simulink model "turbo"  (R2015a)
settings: Solver=ode45  StartTime=0.0  StopTime=10.0  RelTol=1e-3
libraries: commchan3 x4, commdigbbndpm3 x4, commsink2 x2, commcnvcod2 x2, commrandsrc2 x1
settings Model: Creator=jessica.c13  LastModifiedBy=jessica.c13

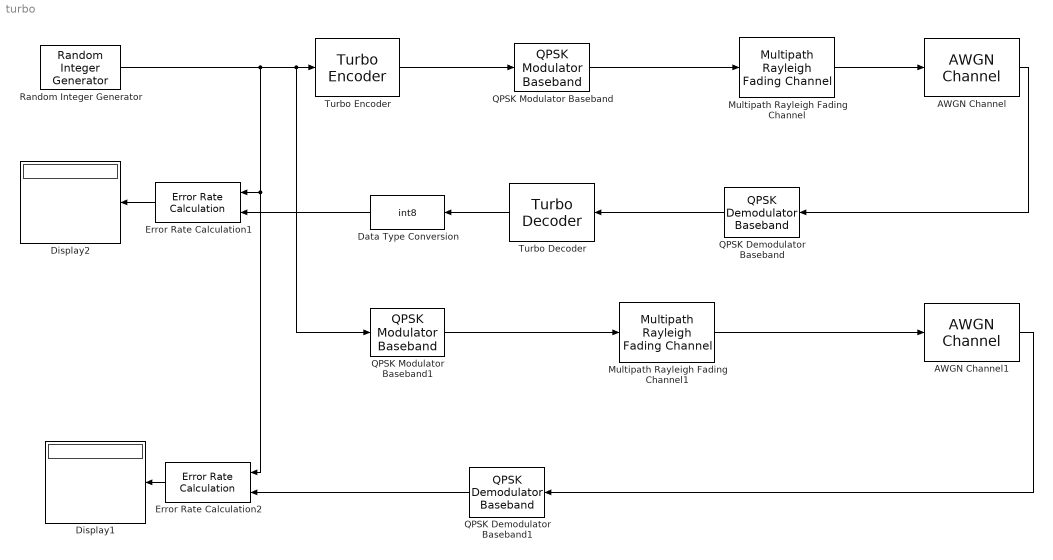
== system turbo ==
  AWGN Channel : commchan3/AWGN Channel  InputProcessing=Columns as channels (frame based)  seed=67  noiseMode="Signal to noise ratio  (Eb/No)"  EbNodB=10  EsNodB=10  SNRdB=10  bitsPerSym=1  Ps=1  Tsym=1  variance=1
  AWGN Channel1 : commchan3/AWGN Channel  InputProcessing=Columns as channels (frame based)  seed=67  noiseMode="Signal to noise ratio  (Eb/No)"  EbNodB=10  EsNodB=10  SNRdB=10  bitsPerSym=1  Ps=1  Tsym=1  variance=1
  Data Type Conversion : DataTypeConversion  OutDataTypeStr=int8
  Display1 : Display
  Display2 : Display
  Error Rate Calculation1 : commsink2/Error Rate Calculation  N=0  st_delay=0  cp_mode=Entire frame  subframe=[]  PMode=Port  WsName=e2  RsMode2=off  stop=off  numErr=100  maxBits=1e6
  Error Rate Calculation2 : commsink2/Error Rate Calculation  N=0  st_delay=0  cp_mode=Entire frame  subframe=[]  PMode=Port  WsName=e2  RsMode2=off  stop=off  numErr=100  maxBits=1e6
  Multipath Rayleigh Fading Channel : commchan3/Multipath Rayleigh Fading Channel  maxDopplerShift=40  spectrumType=Jakes  sigmaGaussian=1/sqrt(2)  coeffRounded=[1 -1.72 0.785]  freqMinMaxRJakes=[0 1]  freqMinMaxAJakes=[0 1]  sigmaGaussian1=1/sqrt(2)  sigmaGaussian2=1/sqrt(2)  centerFreqGaussian1=0.0  centerFreqGaussian2=0.0  gainGaussian1=0.5  gainGaussian2=0.5  coeffBell=9  dopplerSpectrum=doppler.jakes  pathDelays=[0 2e-6]  avgPathGaindB=[0 -3]  normalizePathGains=on  seed=73  enableProbe=0  openVisAtStart=off  outPathGains=off  outDelay=off
  Multipath Rayleigh Fading Channel1 : commchan3/Multipath Rayleigh Fading Channel  maxDopplerShift=40  spectrumType=Jakes  sigmaGaussian=1/sqrt(2)  coeffRounded=[1 -1.72 0.785]  freqMinMaxRJakes=[0 1]  freqMinMaxAJakes=[0 1]  sigmaGaussian1=1/sqrt(2)  sigmaGaussian2=1/sqrt(2)  centerFreqGaussian1=0.0  centerFreqGaussian2=0.0  gainGaussian1=0.5  gainGaussian2=0.5  coeffBell=9  dopplerSpectrum=doppler.jakes  pathDelays=[0 2e-6]  avgPathGaindB=[0 -3]  normalizePathGains=on  seed=73  enableProbe=0  openVisAtStart=off  outPathGains=off  outDelay=off
  QPSK Demodulator Baseband : commdigbbndpm3/QPSK Demodulator Baseband  Ph=pi/4  Dec=Gray  OutType=Integer  DecType=Hard decision  VarSource=Dialog  Variance=1  outDtype1=Inherit via internal rule  outDtype2=double  derotateFactorWordLen=16
  QPSK Demodulator Baseband1 : commdigbbndpm3/QPSK Demodulator Baseband  Ph=pi/4  Dec=Gray  OutType=Integer  DecType=Hard decision  VarSource=Dialog  Variance=1  outDtype1=Inherit via internal rule  outDtype2=int8  derotateFactorWordLen=16
  QPSK Modulator Baseband : commdigbbndpm3/QPSK Modulator Baseband  InType=Integer  Enc=Gray  Ph=pi/4  outDtype=double  outWordLen=16  outUDDataType=sfix(16)  outFracLenMode=Best precision  outFracLen=15
  QPSK Modulator Baseband1 : commdigbbndpm3/QPSK Modulator Baseband  InType=Integer  Enc=Gray  Ph=pi/4  outDtype=double  outWordLen=16  outUDDataType=sfix(16)  outFracLenMode=Best precision  outFracLen=15
  Random Integer Generator : commrandsrc2/Random Integer Generator  mul=2  seed=37  Ts=1/10000  frameBased=on  sampPerFrame=64  orient=off  outDataType=int8
  Turbo Decoder : commcnvcod2/Turbo Decoder  TrellisStructure=poly2trellis( 4, [ 13, 15 ], 13 )  InterleaverIndicesSource=Property  InterleaverIndices=(64:-1:1).'  Algorithm=True APP  NumScalingBits=3  NumIterations=6  SimulateUsing=Interpreted execution
  Turbo Encoder : commcnvcod2/Turbo Encoder  TrellisStructure=poly2trellis( 4, [ 13, 15 ], 13 )  InterleaverIndicesSource=Property  InterleaverIndices=(64:-1:1).'  SimulateUsing=Interpreted execution
  wires:
  Turbo Encoder/1 -> QPSK Modulator Baseband/1
  AWGN Channel/1 -> QPSK Demodulator Baseband/1
  QPSK Demodulator Baseband/1 -> Turbo Decoder/1
  Error Rate Calculation1/1 -> Display2/1
  AWGN Channel1/1 -> QPSK Demodulator Baseband1/1
  Error Rate Calculation2/1 -> Display1/1
  Multipath Rayleigh Fading Channel/1 -> AWGN Channel/1
  Multipath Rayleigh Fading Channel1/1 -> AWGN Channel1/1
  QPSK Modulator Baseband/1 -> Multipath Rayleigh Fading Channel/1
  Random Integer Generator/1 -> Error Rate Calculation1/1, Error Rate Calculation2/1, QPSK Modulator Baseband1/1, Turbo Encoder/1
  QPSK Modulator Baseband1/1 -> Multipath Rayleigh Fading Channel1/1
  QPSK Demodulator Baseband1/1 -> Error Rate Calculation2/2
  Turbo Decoder/1 -> Data Type Conversion/1
  Data Type Conversion/1 -> Error Rate Calculation1/2
